simulink model "Hodgkin"  (Simulink 3.00)
settings: Solver=ode45  SolverMode=SingleTasking  StartTime=0.0  StopTime=18  FixedStep=0.0001  MaxStep=50  RelTol=1e-3
Description:
  | Input parameter
settings Model: InitialStep=10  SaveTime=off  Creator=angel  LastModifiedBy=administrator

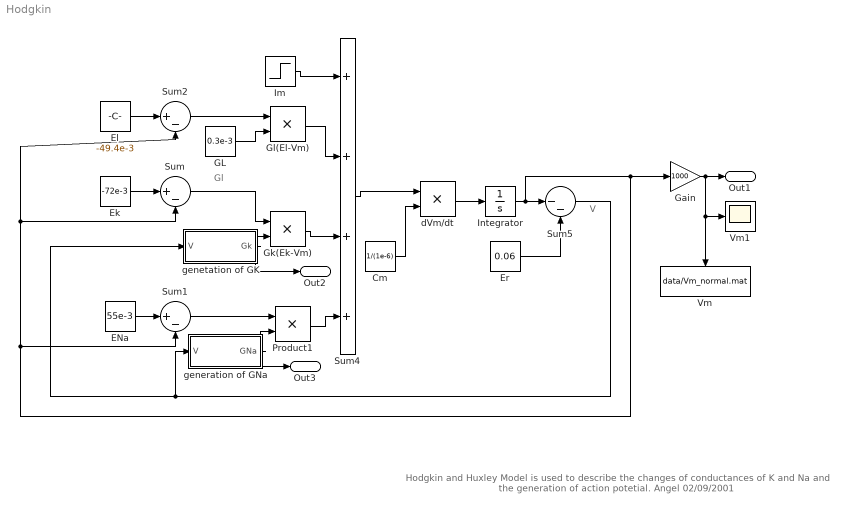
== system Hodgkin ==
  note: Gl
  note: V
  note: Hodgkin and Huxley Model
      | is used to describe the changes of conductances of
      |  K and Na and the generation of  action potetial.
      |                                                       Angel
      |                                                               02/09/2001
  Cm : Constant  Value=1/(1e-6)
  ENa : Constant  Value=55e-3
  Ek : Constant  Value=-72e-3
  El : Constant  Value=-49.4e-3
  Er : Constant  Value=0.06
  GL : Constant  Value=0.3e-3
  Gain : Gain  Gain=1000  SaturateOnIntegerOverflow=on
  Gk(Ek-Vm) : Product  Inputs=2  SaturateOnIntegerOverflow=on
  Gl(El-Vm) : Product  Inputs=2  SaturateOnIntegerOverflow=on
  Im : Step  Time=0  Before=0  After=10e-6  SampleTime=0
  Integrator : Integrator  ExternalReset=none  InitialConditionSource=internal  InitialCondition=-60e-3  LimitOutput=off  UpperSaturationLimit=inf  LowerSaturationLimit=-inf  ShowSaturationPort=off  ShowStatePort=off  AbsoluteTolerance=auto
  Product1 : Product  Inputs=2  SaturateOnIntegerOverflow=on
  Sum : Sum  Inputs=|+-  SaturateOnIntegerOverflow=on
  Sum1 : Sum  Inputs=|+-  SaturateOnIntegerOverflow=on
  Sum2 : Sum  Inputs=|+-  SaturateOnIntegerOverflow=on
  Sum4 : Sum  Inputs=++++  SaturateOnIntegerOverflow=on
  Sum5 : Sum  Inputs=|--  SaturateOnIntegerOverflow=on
  Vm : ToFile  Orientation=down  Filename=data/Vm_normal.mat  MatrixName=Vm  SampleTime=-1
  Vm1 : Scope
      settings: TimeRange=4  YMin=-71  YMax=-65  SaveToWorkspace=off  SaveName=ScopeData
  dVm/dt : Product  Inputs=2  SaturateOnIntegerOverflow=on
  generation of GNa : Subsystem
  genetation of GK : Subsystem
  Out1 : Outport  Port=1
  Out2 : Outport  Port=2
  Out3 : Outport  Port=3
  wires:
  GL/1 -> Gl(El-Vm)/2
  Sum2/1 -> Gl(El-Vm)/1
  Sum4/1 -> dVm/dt/1
  Er/1 -> Sum5/2
  El/1 -> Sum2/1
  Ek/1 -> Sum/1
  Sum/1 -> Gk(Ek-Vm)/1
  ENa/1 -> Sum1/1
  Sum1/1 -> Product1/1
  Cm/1 -> dVm/dt/2
  dVm/dt/1 -> Integrator/1
  Integrator/1 -> Sum5/1, Sum2/2, Sum/2, Sum1/2, Gain/1
  Sum5/1 -> genetation of GK/1(V), generation of GNa/1(V)
  Im/1 -> Sum4/1
  genetation of GK/1(Gk) -> Gk(Ek-Vm)/2, Out2/1
  generation of GNa/1(GNa) -> Product1/2, Out3/1
  Gain/1 -> Vm/1, Vm1/1, Out1/1
  Product1/1 -> Sum4/4
  Gk(Ek-Vm)/1 -> Sum4/3
  Gl(El-Vm)/1 -> Sum4/2

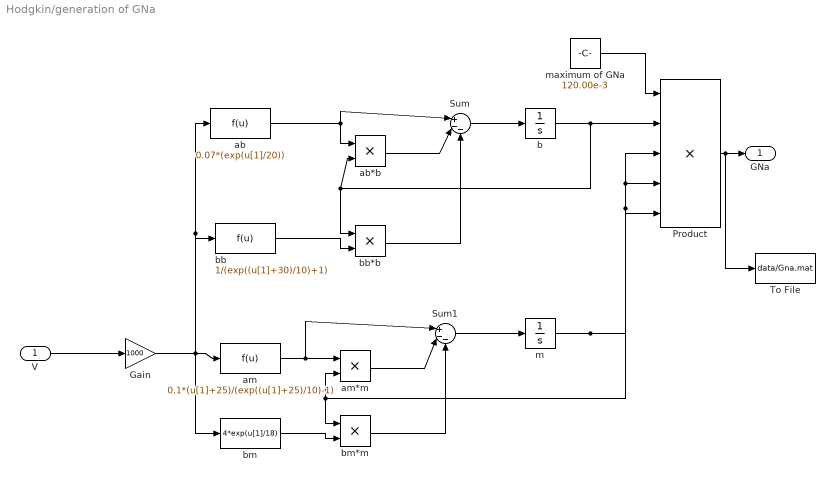
== system Hodgkin/generation of GNa ==
  V : Inport  Port=1  PortWidth=-1  SampleTime=-1  DataType=auto
      settings: SignalType=auto
  Gain : Gain  Gain=1000  SaturateOnIntegerOverflow=on
  Product : Product  Inputs=5  SaturateOnIntegerOverflow=on
  Sum : Sum  Inputs=|+--  SaturateOnIntegerOverflow=on
  Sum1 : Sum  Inputs=|+--  SaturateOnIntegerOverflow=on
  To File : ToFile  Filename=data/Gna.mat  MatrixName=Gna  SampleTime=-1
  ab : Fcn  Expr=0.07*(exp(u[1]/20))
  ab*b : Product  Inputs=2  SaturateOnIntegerOverflow=on
  am : Fcn  Expr=0.1*(u[1]+25)/(exp((u[1]+25)/10)-1)
  am*m : Product  Inputs=2  SaturateOnIntegerOverflow=on
  b : Integrator  ExternalReset=none  InitialConditionSource=internal  InitialCondition=0.59615  LimitOutput=off  UpperSaturationLimit=inf  LowerSaturationLimit=-inf  ShowSaturationPort=off  ShowStatePort=off  AbsoluteTolerance=auto
  bb : Fcn  Expr=1/(exp((u[1]+30)/10)+1)
  bb*b : Product  Inputs=2  SaturateOnIntegerOverflow=on
  bm : Fcn  Expr=4*exp(u[1]/18)
  bm*m : Product  Inputs=2  SaturateOnIntegerOverflow=on
  m : Integrator  ExternalReset=none  InitialConditionSource=internal  InitialCondition=0.05294  LimitOutput=off  UpperSaturationLimit=inf  LowerSaturationLimit=-inf  ShowSaturationPort=off  ShowStatePort=off  AbsoluteTolerance=auto
  maximum of GNa : Constant  Value=120.00e-3
  GNa : Outport  Port=1
  wires:
  bb/1 -> bb*b/2
  ab/1 -> ab*b/1, Sum/1
  ab*b/1 -> Sum/2
  bb*b/1 -> Sum/3
  bm/1 -> bm*m/2
  am*m/1 -> Sum1/2
  bm*m/1 -> Sum1/3
  am/1 -> am*m/1, Sum1/1
  Sum/1 -> b/1
  b/1 -> ab*b/2, bb*b/1, Product/2
  m/1 -> am*m/2, bm*m/1, Product/3, Product/4, Product/5
  maximum of GNa/1 -> Product/1
  Sum1/1 -> m/1
  V/1 -> Gain/1
  Gain/1 -> am/1, ab/1, bb/1, bm/1
  Product/1 -> GNa/1, To File/1

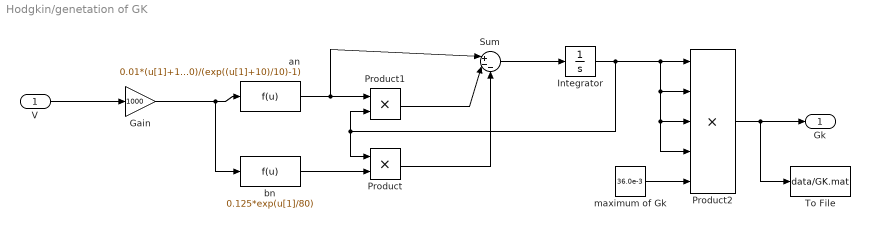
== system Hodgkin/genetation of GK ==
  V : Inport  Port=1  PortWidth=-1  SampleTime=-1  DataType=auto
      settings: SignalType=auto
  Gain : Gain  Gain=1000  SaturateOnIntegerOverflow=on
  Integrator : Integrator  ExternalReset=none  InitialConditionSource=internal  InitialCondition=0.31769  LimitOutput=off  UpperSaturationLimit=inf  LowerSaturationLimit=-inf  ShowSaturationPort=off  ShowStatePort=off  AbsoluteTolerance=auto
  Product : Product  Inputs=2  SaturateOnIntegerOverflow=on
  Product1 : Product  Inputs=2  SaturateOnIntegerOverflow=on
  Product2 : Product  Inputs=5  SaturateOnIntegerOverflow=on
  Sum : Sum  Inputs=|+--  SaturateOnIntegerOverflow=on
  To File : ToFile  Filename=data/GK.mat  MatrixName=Gk  SampleTime=-1
  an : Fcn  Expr=0.01*(u[1]+10)/(exp((u[1]+10)/10)-1)
  bn : Fcn  Expr=0.125*exp(u[1]/80)
  maximum of Gk : Constant  Value=36.0e-3
  Gk : Outport  Port=1
  wires:
  bn/1 -> Product/2
  an/1 -> Product1/1, Sum/1
  Product1/1 -> Sum/2
  Product/1 -> Sum/3
  Sum/1 -> Integrator/1
  Integrator/1 -> Product1/2, Product/1, Product2/1, Product2/2, Product2/3, Product2/4
  maximum of Gk/1 -> Product2/5
  V/1 -> Gain/1
  Gain/1 -> an/1, bn/1
  Product2/1 -> Gk/1, To File/1
